simulink model "quad_quaternion_tracking"  (R2025b)
settings: Solver=VariableStepAuto  StartTime=0.0  StopTime=10.0  RelTol=1e-3
values from neighbouring files (symbols this model uses):
  g = 9.81    [init_params.m]
  m = 0.025    [init_params.m]
undefined symbols (not defined in the file or in its folder): kq
libraries: aerolibutil x2
settings Model: Creator=ASUS  LastModifiedBy=ASUS

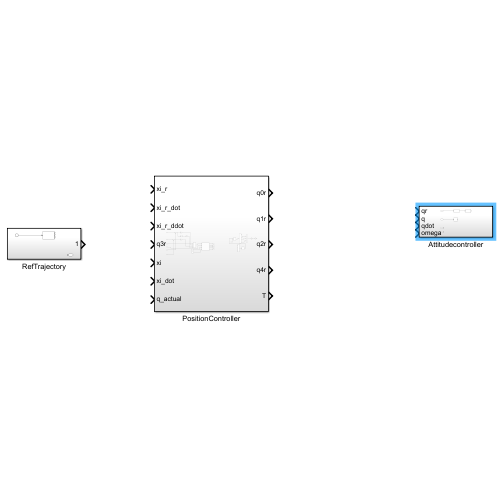
[thumbnail: Simulink's stored preview of the top-level diagram]
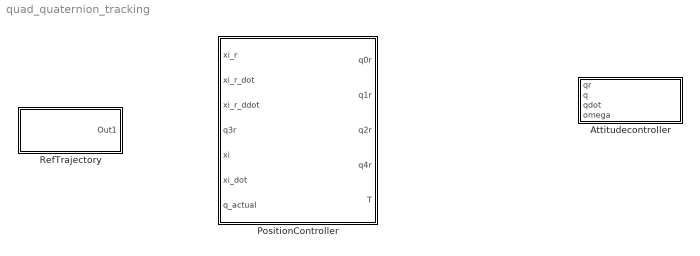
== system quad_quaternion_tracking ==
  Attitudecontroller : Subsystem
  PositionController : Subsystem
  RefTrajectory : Subsystem

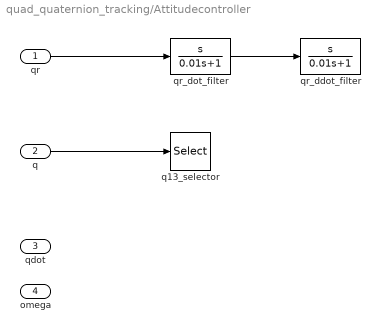
== system quad_quaternion_tracking/Attitudecontroller ==
  qr : Inport
  q : Inport  Port=2
  qdot : Inport  Port=3
  omega : Inport  Port=4
  q13_selector : Selector  InputPortWidth=3  IndexOptions=Index vector (dialog)  Indices=[1 3]  OutputSizes=1
  qr_ddot_filter : TransferFcn  Numerator=[1 0]  Denominator=[0.01 1]
  qr_dot_filter : TransferFcn  Numerator=[1 0]  Denominator=[0.01 1]
  wires:
  qr/1 -> qr_dot_filter/1
  qr_dot_filter/1 -> qr_ddot_filter/1
  q/1 -> q13_selector/1

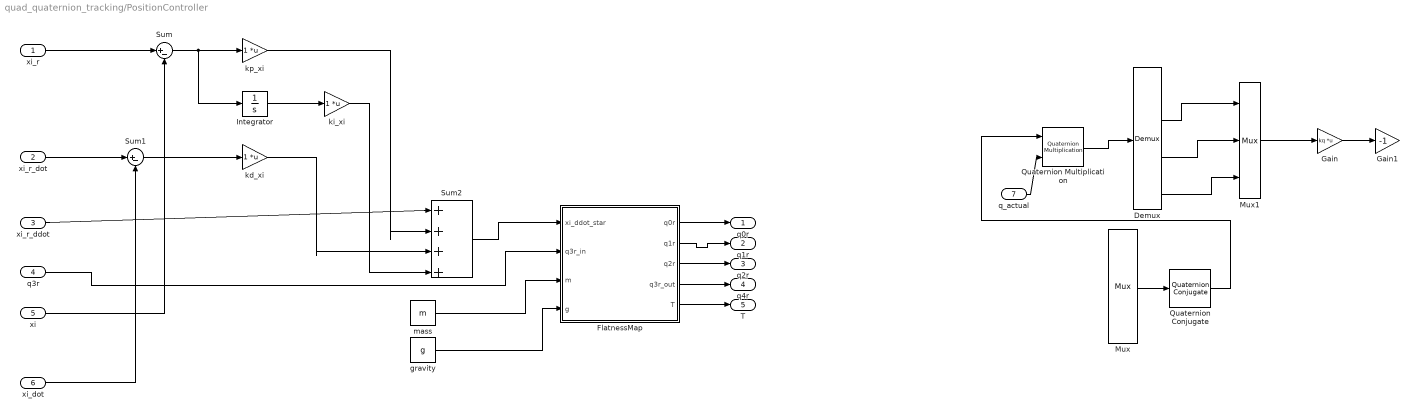
== system quad_quaternion_tracking/PositionController ==
  xi_r : Inport
  xi_r_dot : Inport  Port=2
  xi_r_ddot : Inport  Port=3
  q3r : Inport  Port=4
  xi : Inport  Port=5
  xi_dot : Inport  Port=6
  q_actual : Inport  Port=7
  Demux : Demux
  FlatnessMap : MATLAB Function  TreatAsAtomicUnit=on
  Gain : Gain  Gain=kq  Multiplication=Matrix(K*u)
  Gain1 : Gain  Gain=-1
  Integrator : Integrator
  Mux : Mux
  Mux1 : Mux  Inputs=3
  Quaternion Conjugate : aerolibutil/Quaternion Conjugate
  Quaternion Multiplication : aerolibutil/Quaternion Multiplication
  Sum : Sum  Inputs=|+-
  Sum1 : Sum  Inputs=|+-
  Sum2 : Sum  Inputs=|++++
  gravity : Constant  Value=g
  kd_xi : Gain  Multiplication=Matrix(K*u)
  "ki_xi " : Gain  Multiplication=Matrix(K*u)
  kp_xi : Gain  Multiplication=Matrix(K*u)
  mass : Constant  Value=m
  q0r : Outport  VectorParamsAs1DForOutWhenUnconnected=off
  q1r : Outport  Port=2  VectorParamsAs1DForOutWhenUnconnected=off
  q2r : Outport  Port=3  VectorParamsAs1DForOutWhenUnconnected=off
  q4r : Outport  Port=4  VectorParamsAs1DForOutWhenUnconnected=off
  T : Outport  Port=5  VectorParamsAs1DForOutWhenUnconnected=off
  wires:
  xi_r/1 -> Sum/1
  xi/1 -> Sum/2
  Integrator/1 -> "ki_xi "/1
  kp_xi/1 -> Sum2/2
  xi_r_dot/1 -> Sum1/1
  xi_dot/1 -> Sum1/2
  Sum1/1 -> kd_xi/1
  xi_r_ddot/1 -> Sum2/1
  kd_xi/1 -> Sum2/3
  Sum/1 -> Integrator/1, kp_xi/1
  "ki_xi "/1 -> Sum2/4
  Sum2/1 -> FlatnessMap/1(xi_ddot_star)
  q3r/1 -> FlatnessMap/2(q3r_in)
  mass/1 -> FlatnessMap/3(m)
  gravity/1 -> FlatnessMap/4(g)
  FlatnessMap/1(q0r) -> q0r/1
  FlatnessMap/2(q1r) -> q1r/1
  FlatnessMap/3(q2r) -> q2r/1
  FlatnessMap/4(q3r_out) -> q4r/1
  FlatnessMap/5(T) -> T/1
  Mux/1 -> Quaternion Conjugate/1
  Quaternion Conjugate/1 -> Quaternion Multiplication/1
  Quaternion Multiplication/1 -> Demux/1
  q_actual/1 -> Quaternion Multiplication/2
  Demux/2 -> Mux1/1
  Demux/3 -> Mux1/2
  Demux/4 -> Mux1/3
  Mux1/1 -> Gain/1
  Gain/1 -> Gain1/1

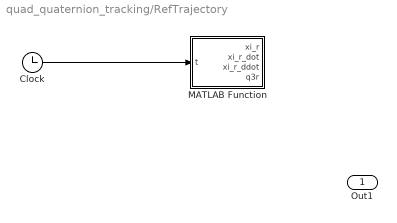
== system quad_quaternion_tracking/RefTrajectory ==
  Clock : Clock
  MATLAB Function : MATLAB Function  TreatAsAtomicUnit=on
  Out1 : Outport
  wires:
  Clock/1 -> MATLAB Function/1(t)

== matlab function quad_quaternion_tracking/RefTrajectory/MATLAB Function ==
  data: t input; xi_r output; xi_r_dot output; xi_r_ddot output; q3r output
function [xi_r, xi_r_dot, xi_r_ddot, q3r] = RefTrajectory(t)

% Waypoints
p0 = [1.8; 2.27; 0.6];
t0 = 0;

p1 = [2.9; 3; 1.2];
t1 = 6;

p2 = [2.9; 3; 1.2];
t2 = 14;

p3 = [3.6; 2; 0.6];
t3 = 20;

if t <= t1

    [xi_r, xi_r_dot, xi_r_ddot] = ...
        quinticSeg(t,t0,t1,p0,p1);

elseif t <= t2

    xi_r = p1;
    xi_r_dot = [0;0;0];
    xi_r_ddot = [0;0;0];

else

    [xi_r, xi_r_dot, xi_r_ddot] = ...
        quinticSeg(t,t2,t3,p2,p3);

end

q3r = 0;

end


function [p,v,a] = quinticSeg(t,ta,tb,pa,pb)

T = tb-ta;

tau = min(max((t-ta)/T,0),1);

s = 10*tau.^3 ...
    - 15*tau.^4 ...
    + 6*tau.^5;

sd = (30*tau.^2 ...
    - 60*tau.^3 ...
    + 30*tau.^4)/T;

sdd = (60*tau ...
    - 180*tau.^2 ...
    + 120*tau.^3)/T^2;

p = pa + (pb-pa).*s;

v = (pb-pa).*sd;

a = (pb-pa).*sdd;

end

== matlab function quad_quaternion_tracking/PositionController/FlatnessMap ==
  data: xi_ddot_star input; q0r output; q3r_in input; m input; g input; q1r output; q2r output; q3r_out output; T output
function [q0r,q1r,q2r,q3r_out,T] = FlatnessMap(xi_ddot_star,q3r_in,m,g)

xdd = xi_ddot_star(1);
ydd = xi_ddot_star(2);
zdd = xi_ddot_star(3);

normA = sqrt(xdd^2 + ydd^2 + (zdd+g)^2);

T = m*normA;

q3r_out = q3r_in;

inner = (zdd+g)/normA - 2*q3r_in^2 + 1;

inner = max(inner,0);

sq = sqrt(inner);

q0r = (1/sqrt(2))*sq;

denom = (zdd+g) + normA;

denom = sign(denom)*max(abs(denom),1e-6);

q1r = (xdd*q3r_in - (1/sqrt(2))*ydd*sq)/denom;

q2r = (ydd*q3r_in + (1/sqrt(2))*xdd*sq)/denom;

end
